simulink model "untitled"  (R2012b)
settings: Solver=ode45  StartTime=0.0  StopTime=10.0  RelTol=1e-3
settings Model: Creator=Henrique.Alles  LastModifiedBy=Henrique.Alles

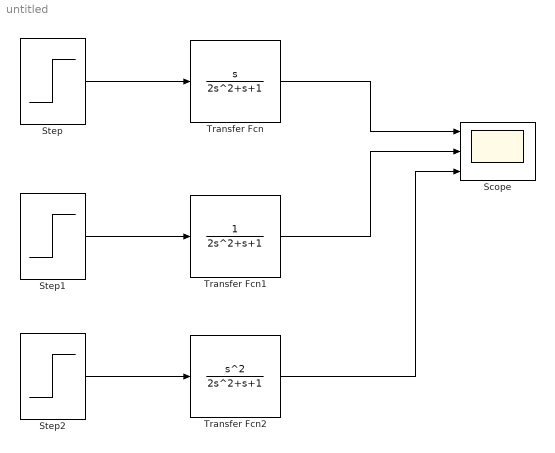
== system untitled ==
  Scope : Scope  NumInputPorts=3
      settings: YMin=-5~-5~-5  YMax=5~5~5
  Step : Step  After=3  SampleTime=0
  Step1 : Step  After=3  SampleTime=0
  Step2 : Step  After=3  SampleTime=0
  Transfer Fcn : TransferFcn  Numerator=[1 0]  Denominator=[2 1 1]
  Transfer Fcn1 : TransferFcn  Denominator=[2 1 1]
  Transfer Fcn2 : TransferFcn  Numerator=[1 0 0]  Denominator=[2 1 1]
  wires:
  Step/1 -> Transfer Fcn/1
  Transfer Fcn/1 -> Scope/1
  Step1/1 -> Transfer Fcn1/1
  Transfer Fcn1/1 -> Scope/2
  Step2/1 -> Transfer Fcn2/1
  Transfer Fcn2/1 -> Scope/3
